simulink model "AnalyticalOrbitPropagator"  (R2023a)
settings: Solver=ode4  StartTime=0.0  StopTime=10.0  FixedStep=600  RelTol=1e-3
settings Model: Creator=ndelurgio  LastModifiedBy=ndelurgio

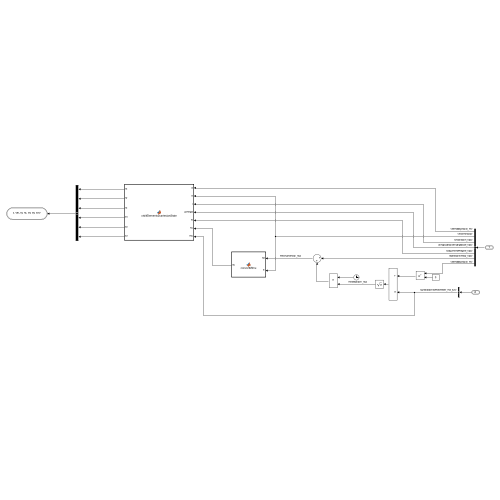
[thumbnail: Simulink's stored preview of the top-level diagram]
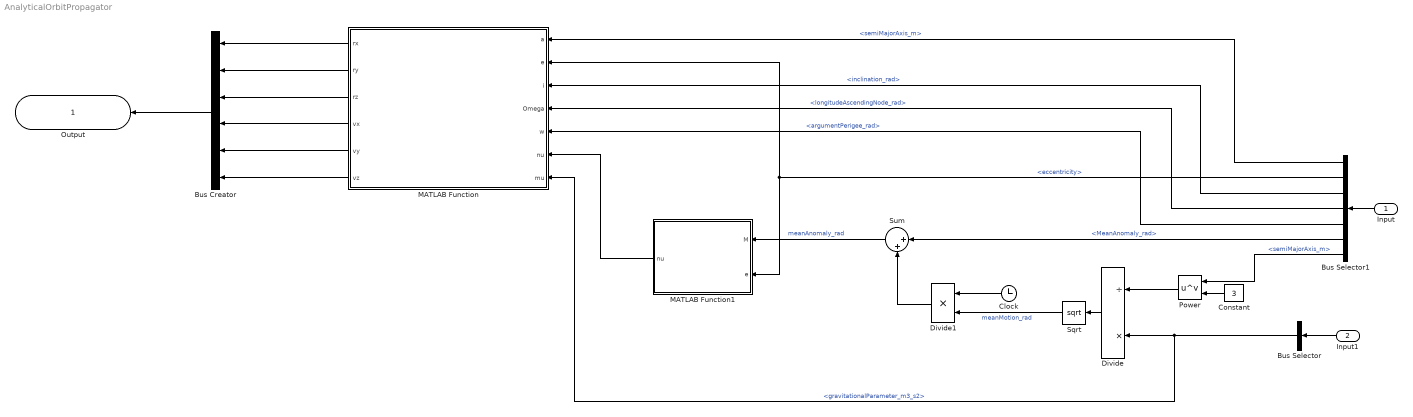
== system AnalyticalOrbitPropagator ==
  Input : Inport  OutDataTypeStr=Bus: orbitElements
  Input1 : Inport  Port=2  OutDataTypeStr=Bus: earthProperties
  Bus Creator : BusCreator  Inputs=6  OutDataTypeStr=Bus: cartesianState  NonVirtualBus=on
      settings: InheritFromInputs=off
  Bus Selector : BusSelector  OutputSignals=gravitationalParameter_m3_s2
  Bus Selector1 : BusSelector  OutputSignals=semiMajorAxis_m,eccentricity,inclination_rad,longitudeAscendingNode_rad,argumentPerigee_rad,MeanAnomaly_rad,semiMajorAxis_m
  Clock : Clock
  Constant : Constant  Value=3
  Divide : Product  Inputs=/*
  Divide1 : Product  Inputs=**
  MATLAB Function : MATLAB Function  TreatAsAtomicUnit=on
  MATLAB Function1 : MATLAB Function  TreatAsAtomicUnit=on
  Power : Math  Operator=pow
  Sqrt : Sqrt
  Sum : Sum  Inputs=|++
  Output : Outport  OutDataTypeStr=Bus: cartesianState  BusOutputAsStruct=on
  wires:
  Input1/1 -> Bus Selector/1
  Bus Selector/1 -> MATLAB Function/7(mu), Divide/2  "<gravitationalParameter_m3_s2>"
  Input/1 -> Bus Selector1/1
  Bus Selector1/6 -> Sum/1  "<MeanAnomaly_rad>"
  Constant/1 -> Power/2
  Power/1 -> Divide/1
  Divide/1 -> Sqrt/1
  Sqrt/1 -> Divide1/2  "meanMotion_rad"
  Clock/1 -> Divide1/1
  Divide1/1 -> Sum/2
  Sum/1 -> MATLAB Function1/1(M)  "meanAnomaly_rad"
  Bus Selector1/7 -> Power/1  "<semiMajorAxis_m>"
  Bus Selector1/5 -> MATLAB Function/5(w)  "<argumentPerigee_rad>"
  Bus Selector1/4 -> MATLAB Function/4(Omega)  "<longitudeAscendingNode_rad>"
  Bus Selector1/3 -> MATLAB Function/3(i)  "<inclination_rad>"
  Bus Selector1/2 -> MATLAB Function1/2(e), MATLAB Function/2(e)  "<eccentricity>"
  Bus Selector1/1 -> MATLAB Function/1(a)  "<semiMajorAxis_m>"
  MATLAB Function1/1(nu) -> MATLAB Function/6(nu)
  MATLAB Function/1(rx) -> Bus Creator/1
  MATLAB Function/2(ry) -> Bus Creator/2
  MATLAB Function/3(rz) -> Bus Creator/3
  MATLAB Function/4(vx) -> Bus Creator/4
  MATLAB Function/5(vy) -> Bus Creator/5
  MATLAB Function/6(vz) -> Bus Creator/6
  Bus Creator/1 -> Output/1

== matlab function AnalyticalOrbitPropagator/MATLAB Function1 ==
  data: M input; nu output; e input
function nu = convertM2nu(M,e)
nu = M2nu(M,e);
end

== matlab function AnalyticalOrbitPropagator/MATLAB Function ==
  data: a input; rx output; e input; i input; Omega input; w input; nu input; ry output; rz output; vx output; vy output; vz output; mu input
function [rx,ry,rz,vx,vy,vz] = orbitElements2cartesianState(a,e,i,Omega,w,nu,mu)

% coder.extrinsic("keplerian2ijk")
[r_eci, v_eci] = oe2eci(a,e,i,Omega,w,nu,mu);

rx = r_eci(1);
ry = r_eci(2);
rz = r_eci(3);

vx = v_eci(1);
vy = v_eci(2);
vz = v_eci(3);

end
